simulink model "sfcndemo_sdotproduct"  (Simulink 7.6)
settings: Solver=FixedStepDiscrete  StartTime=0.0  StopTime=5.0  FixedStep=1  RelTol=1e-3
Description:
  | Compute Dot Product (Multiply-Accumulate) with C-MEX S-function
settings Model: Creator=The MathWorks Inc.  ExtModeTrigMode=oneshot  ExtModeArmWhenConnect=off  ExtModeAutoUpdateStatusClock=off
settings DataIOCC: LimitDataPoints=off
settings OptimizationCC: BooleanDataType=off  InlineInvariantSignals=on  InitFltsAndDblsToZero=on
settings DebuggingCC: SaveWithParameterizedLinksMsg=none  SignalResolutionControl=TryResolveAllWithWarning  SolverPrmCheckMsg=none  MultiTaskDSMMsg=warning  MultiTaskCondExecSysMsg=none
settings HardwareCC: TargetUnknown=on
settings RTWCC: IncludeERTFirstTime=on
settings CodeAppCC: CustomSymbolStrFcn=$F$N$M
settings GRTTargetCC: TargetFcnLib=ansi_tfl_tmw.mat

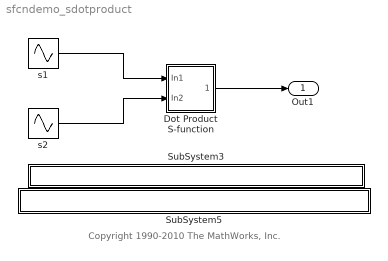
== system sfcndemo_sdotproduct ==
  note: Copyright 1990-2010 The MathWorks, Inc.
  Dot Product S-function : Subsystem  mask(S-function: Dot Product){}
      mask help:
      | Inner (dot) product.
      | y=sum(u1.*u2)
      mask init:
      | t=(0:.1:2*pi)';
      | x=cos(t);
      | y=sin(t);
      | r=0.05;
      mask Help: Computes the inner (dot) product of the inputs: sum(u1.*u2).  The inputs are vectors of the same length. Output is a scalar.
      mask Display: patch([x*r+0.5],[y*r+0.5]);disp('\n\ns-func');
  SubSystem3 : Subsystem  mask{filename=sdotproduct.c}
      mask init:
      | x=sfundemo_maskdisp;
      settings: AttributesFormatString=\n  OpenFcn=sfundemo_openfcn
      mask Display: disp(x);
  SubSystem5 : Subsystem  mask{filename=sdotproduct.tlc}
      mask init:
      | x=sfundemo_maskdisp;
      settings: AttributesFormatString=\n  OpenFcn=sfundemo_openfcn
      mask Display: disp(x);
  s1 : Sin  Amplitude=[1:20]  SampleTime=0
  s2 : Sin  Amplitude=21:40  Phase=pi/2  SampleTime=0
  Out1 : Outport
  wires:
  s2/1 -> Dot Product S-function/2(In2)
  s1/1 -> Dot Product S-function/1(In1)
  Dot Product S-function/1(Out1) -> Out1/1

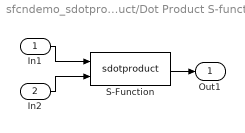
== system sfcndemo_sdotproduct/Dot Product S-function ==
  In1 : Inport
  In2 : Inport  Port=2
  S-Function : S-Function  FunctionName=sdotproduct  EnableBusSupport=off
  Out1 : Outport
  wires:
  In2/1 -> S-Function/2
  In1/1 -> S-Function/1
  S-Function/1 -> Out1/1

== system sfcndemo_sdotproduct/SubSystem3 ==

== system sfcndemo_sdotproduct/SubSystem5 ==
